simulink model "Iteration_1"  (R2025b)
settings: Solver=VariableStepAuto  StartTime=0.0  StopTime=15  RelTol=1e-3
values from neighbouring files (symbols this model uses):
  A = [ -(Cf + Cr)/(m*vx),            ((lr*Cr - lf*Cf)/(m*vx)) - vx,   0,   0 ... (first row only)    [Init_Script.m]    (also in lka_phase3_results.mat = [0  20; 0  0])
  B = [ Cf/m ... (first row only)    [Init_Script.m]    (also in lka_phase3_results.mat = [0 7.40740740741])
  Bc = [0; 0; 0; -1]    [Init_Script.m]
  Bd = [1/m; 0; 0; 0]    [Init_Script.m]
  K = [10 8]    [lka_phase3_results.mat]
  x0 = [0; 0; 0.3; 0.05]    [Init_Script.m]    (also in lka_phase3_results.mat = [0.3 0.05])
libraries: simulink x3
settings Model: Creator=Ayan  LastModifiedBy=Ayan

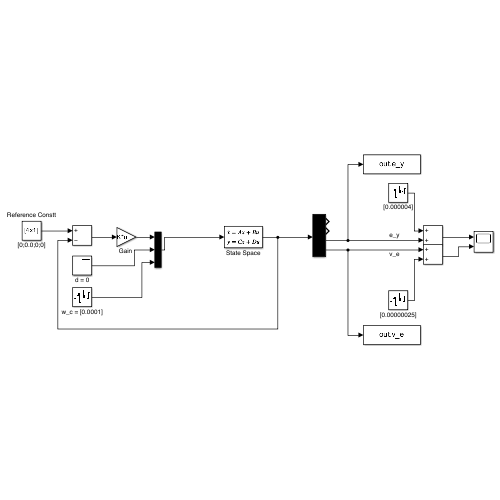
[thumbnail: Simulink's stored preview of the top-level diagram]
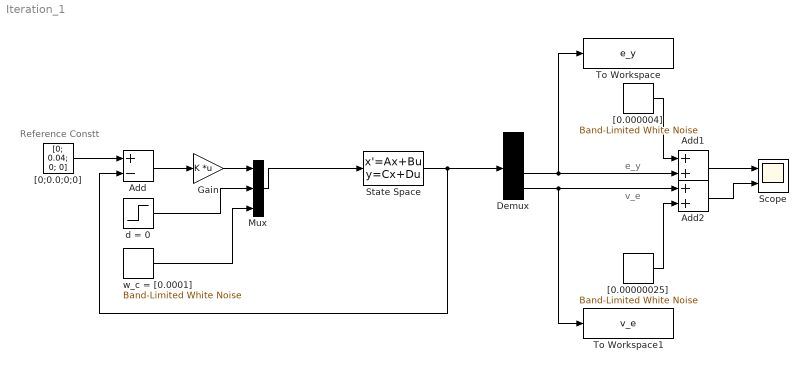
== system Iteration_1 ==
  note: Reference Constt
  note: v_e
  note: e_y
  Add : Sum  Inputs=+-
  Add1 : Sum
  Add2 : Sum
  Demux : Demux
  "Gain " : Gain  Gain=K  Multiplication=Matrix(K*u)
  Mux : Mux  Inputs=3
  Scope : Scope  NumInputPorts=2
      settings: ActiveDisplayYMinimum=-0.29869221678405544  ActiveDisplayYMaximum=0.35644424173048828
  State Space : StateSpace  A=A  B=[B, Bd, Bc]  C=eye(4)  D=zeros(4, 3)  InitialCondition=x0
  To Workspace : ToWorkspace  VariableName=e_y  SampleTime=-1
  To Workspace1 : ToWorkspace  VariableName=v_e  SampleTime=-1
  "[0.00000025]" : simulink/Sources/Band-Limited White Noise  Cov=[0.00000025]  Ts=0.033  seed=[23341]
  "[0.000004]" : simulink/Sources/Band-Limited White Noise  Cov=[0.000004]  Ts=0.033  seed=[23341]
  "[0;0.0;0;0]" : Constant  Value=[0; 0.04; 0; 0]
  d = 0 : Step  Time=5  After=0  SampleTime=0
  w_c = [0.0001] : simulink/Sources/Band-Limited White Noise  Cov=[0.0001]  Ts=0.1  seed=[23341]
  wires:
  "[0;0.0;0;0]"/1 -> Add/1
  Add/1 -> "Gain "/1
  State Space/1 -> Demux/1, Add/2
  Demux/4 -> To Workspace1/1, Add2/1
  Demux/3 -> To Workspace/1, Add1/2
  "[0.000004]"/1 -> Add1/1
  "[0.00000025]"/1 -> Add2/2
  "Gain "/1 -> Mux/1
  Mux/1 -> State Space/1
  d = 0/1 -> Mux/2
  w_c = [0.0001]/1 -> Mux/3
  Add1/1 -> Scope/1
  Add2/1 -> Scope/2
